simulink model "V2"  (R2022b)
settings: Solver=VariableStepAuto  StartTime=0.0  StopTime=30  RelTol=1e-3
libraries: simulink x4
settings Model: Creator=rrilo  LastModifiedBy=rrilo

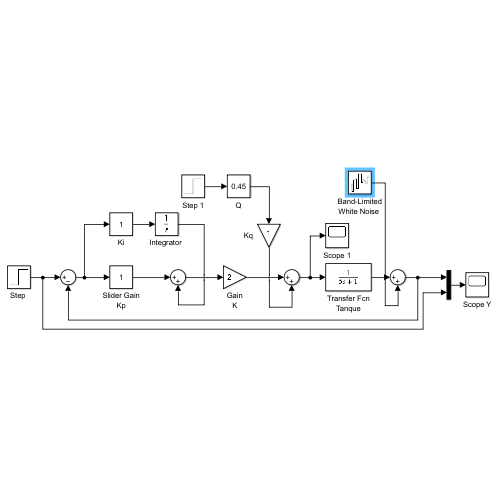
[thumbnail: Simulink's stored preview of the top-level diagram]
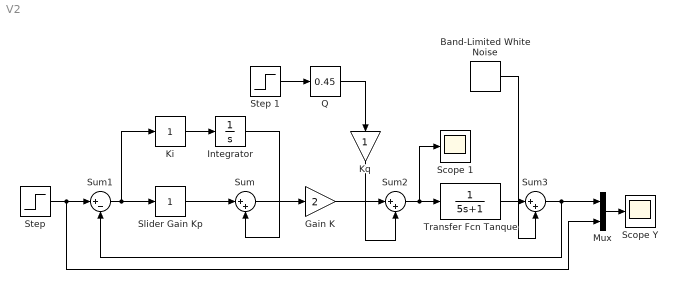
== system V2 ==
  "Band-Limited White Noise " : simulink/Sources/Band-Limited White Noise  Cov=[0]  Ts=0.1  seed=[23341]
  Gain K : Gain  Gain=2
  "Integrator " : Integrator
  Ki : simulink/Math Operations/Slider Gain  gain=1  low=0  high=20
  Kq : Gain
  Mux : Mux  Inputs=2
  Q : simulink/Math Operations/Slider Gain  gain=0.45  low=0  high=1
  Scope 1 : Scope
  Scope Y : Scope
  Slider Gain Kp : simulink/Math Operations/Slider Gain  gain=1  low=0  high=20
  "Step " : Step  SampleTime=0
  Step 1 : Step  SampleTime=20
  Sum : Sum  Inputs=|++
  Sum1 : Sum  Inputs=|+-
  Sum2 : Sum  Inputs=|++
  Sum3 : Sum  Inputs=|++
  Transfer Fcn Tanque : TransferFcn  Denominator=[5 1]
  wires:
  Mux/1 -> Scope Y/1
  Sum2/1 -> Scope 1/1, Transfer Fcn Tanque/1
  Step 1/1 -> Q/1
  Kq/1 -> Sum2/2
  Sum/1 -> Gain K/1
  Slider Gain Kp/1 -> Sum/1
  Sum1/1 -> Ki/1, Slider Gain Kp/1
  Q/1 -> Kq/1
  "Integrator "/1 -> Sum/2
  Gain K/1 -> Sum2/1
  "Step "/1 -> Mux/2, Sum1/1
  "Band-Limited White Noise "/1 -> Sum3/2
  Transfer Fcn Tanque/1 -> Sum3/1
  Sum3/1 -> Sum1/2, Mux/1
  Ki/1 -> "Integrator "/1
